simulink model "featureExtractionTest"  (R2021a)
settings: Solver=FixedStepDiscrete  StartTime=0.0  StopTime=stopTime  RelTol=1e-3
PostLoadFcn:
  | addpath([fileparts(which(bdroot)) filesep '..' filesep])
InitFcn:
  | simulinkInitFeatureExtraction
StopFcn:
  | simulinkVerifyFeatureExtraction
undefined symbols (not defined in the file or in its folder): params
libraries: hdlsllib x10, dspsrcs4 x1
settings Model: DataTypeOverride=Off  SimulationMode=accelerator  PauseTimes=1  Creator=trevor  LastModifiedBy=trevvvy
settings SolverCC: AlgebraicLoopSolver=TrustRegion
settings DataIOCC: SaveFormat=Array  SaveOutput=off  DSMLogging=off  SaveTime=off  ReturnWorkspaceOutputs=off
settings OptimizationCC: BlockReduction=off  ConditionallyExecuteInputs=off  DefaultParameterBehavior=Inlined
settings DebuggingCC: AlgebraicLoopMsg=error  SingleTaskRateTransMsg=error
settings HardwareCC: ProdBitPerPointer=32  ProdBitPerSizeT=32  ProdBitPerPtrDiffT=32  ProdLargestAtomicFloat=None  ProdIntDivRoundTo=Undefined  ProdEndianess=Unspecified  ProdWordSize=32  ProdHWDeviceType=ASIC/FPGA->ASIC/FPGA  TargetBitPerLong=64  TargetBitPerPointer=64  TargetBitPerSizeT=64  TargetBitPerPtrDiffT=64  TargetLongLongMode=on  TargetIntDivRoundTo=Zero  TargetEndianess=LittleEndian  TargetWordSize=64  TargetHWDeviceType=Custom Processor->MATLAB Host Computer  ProdEqTarget=off

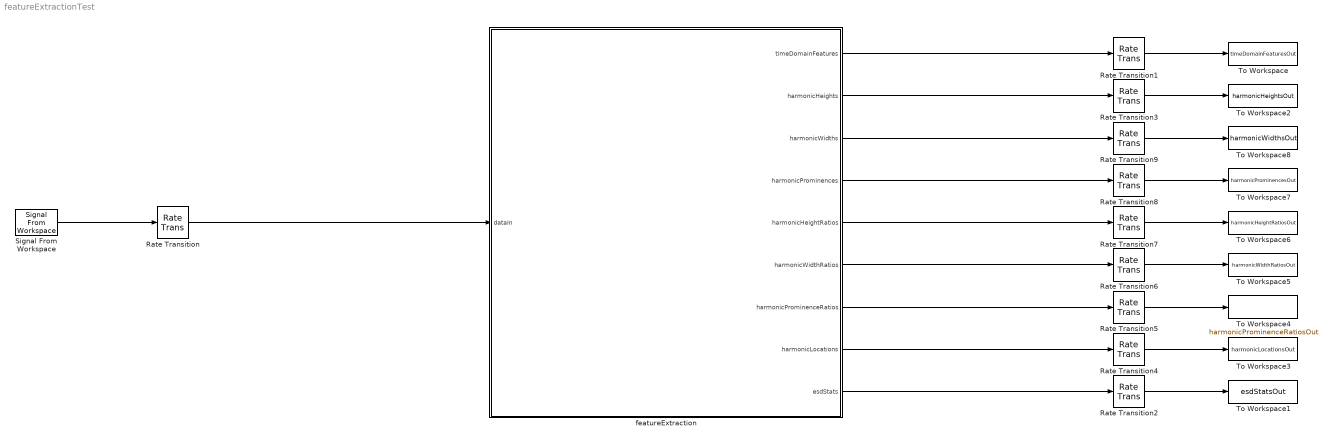
== system featureExtractionTest ==
  Rate Transition : RateTransition  Deterministic=off  OutPortSampleTime=params.systemClockPeriod
  Rate Transition{1..9} (9 alike) : RateTransition  OutPortSampleTime=params.samplingPeriod
  Signal From Workspace : dspsrcs4/Signal From Workspace  X=testData  Ts=params.samplingPeriod  nsamps=1  OutputAfterFinalValue=Setting to zero  ignoreOrWarnInputAndFrameLengths=off  OutputFrames=off
  To Workspace : ToWorkspace  VariableName=timeDomainFeaturesOut  SampleTime=-1
      settings: Save2DSignal=2-D array (concatenate along first dimension)
  To Workspace1 : ToWorkspace  VariableName=esdStatsOut  SampleTime=-1
      settings: Save2DSignal=2-D array (concatenate along first dimension)
  To Workspace2 : ToWorkspace  VariableName=harmonicHeightsOut  SampleTime=-1
      settings: Save2DSignal=2-D array (concatenate along first dimension)
  To Workspace3 : ToWorkspace  VariableName=harmonicLocationsOut  SampleTime=-1
      settings: Save2DSignal=2-D array (concatenate along first dimension)
  To Workspace4 : ToWorkspace  VariableName=harmonicProminenceRatiosOut  SampleTime=-1
      settings: Save2DSignal=2-D array (concatenate along first dimension)
  To Workspace5 : ToWorkspace  VariableName=harmonicWidthRatiosOut  SampleTime=-1
      settings: Save2DSignal=2-D array (concatenate along first dimension)
  To Workspace6 : ToWorkspace  VariableName=harmonicHeightRatiosOut  SampleTime=-1
      settings: Save2DSignal=2-D array (concatenate along first dimension)
  To Workspace7 : ToWorkspace  VariableName=harmonicProminencesOut  SampleTime=-1
      settings: Save2DSignal=2-D array (concatenate along first dimension)
  To Workspace8 : ToWorkspace  VariableName=harmonicWidthsOut  SampleTime=-1
      settings: Save2DSignal=2-D array (concatenate along first dimension)
  featureExtraction : Subsystem
  wires:
  Signal From Workspace/1 -> Rate Transition/1
  Rate Transition1/1 -> To Workspace/1
  Rate Transition2/1 -> To Workspace1/1
  Rate Transition3/1 -> To Workspace2/1
  Rate Transition4/1 -> To Workspace3/1
  Rate Transition5/1 -> To Workspace4/1
  Rate Transition6/1 -> To Workspace5/1
  Rate Transition7/1 -> To Workspace6/1
  Rate Transition9/1 -> To Workspace8/1
  Rate Transition8/1 -> To Workspace7/1
  Rate Transition/1 -> featureExtraction/1(dataIn)
  featureExtraction/1(timeDomainFeatures) -> Rate Transition1/1
  featureExtraction/2(harmonicHeights) -> Rate Transition3/1
  featureExtraction/3(harmonicWidths) -> Rate Transition9/1
  featureExtraction/4(harmonicProminences) -> Rate Transition8/1
  featureExtraction/5(harmonicHeightRatios) -> Rate Transition7/1
  featureExtraction/6(harmonicWidthRatios) -> Rate Transition6/1
  featureExtraction/7(harmonicProminenceRatios) -> Rate Transition5/1
  featureExtraction/8(harmonicLocations) -> Rate Transition4/1
  featureExtraction/9(esdStats) -> Rate Transition2/1

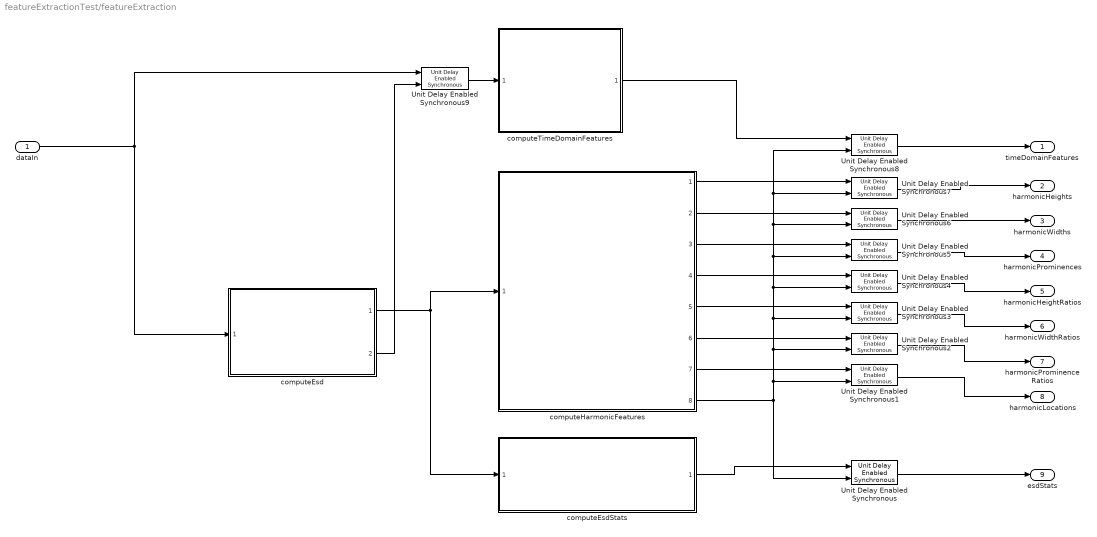
== system featureExtractionTest/featureExtraction ==
  dataIn : Inport
  Unit Delay Enabled Synchronous{,1..9} (10 alike) : hdlsllib/Discrete/Unit Delay Enabled Synchronous  InitialCondition=0.0  SampleTime=-1
      settings: SourceProductBaseCode=SL
  computeEsd : Subsystem  ReferencedSubsystem=ESD
  computeEsdStats : Subsystem  ReferencedSubsystem=extractEsdStats
  computeHarmonicFeatures : Subsystem  ReferencedSubsystem=harmonicFeatures
  computeTimeDomainFeatures : Subsystem  ReferencedSubsystem=timeDomainFeatures
  timeDomainFeatures : Outport
  harmonicHeights : Outport  Port=2
  harmonicWidths : Outport  Port=3
  harmonicProminences : Outport  Port=4
  harmonicHeightRatios : Outport  Port=5
  harmonicWidthRatios : Outport  Port=6
  harmonicProminenceRatios : Outport  Port=7
  harmonicLocations : Outport  Port=8
  esdStats : Outport  Port=9
  wires:
  computeHarmonicFeatures/6 -> Unit Delay Enabled Synchronous2/1
  Unit Delay Enabled Synchronous3/1 -> harmonicWidthRatios/1
  Unit Delay Enabled Synchronous8/1 -> timeDomainFeatures/1
  computeEsd/1 -> computeEsdStats/1, computeHarmonicFeatures/1
  computeTimeDomainFeatures/1 -> Unit Delay Enabled Synchronous8/1
  computeHarmonicFeatures/7 -> Unit Delay Enabled Synchronous1/1
  computeHarmonicFeatures/5 -> Unit Delay Enabled Synchronous3/1
  dataIn/1 -> computeEsd/1, Unit Delay Enabled Synchronous9/1
  Unit Delay Enabled Synchronous7/1 -> harmonicHeights/1
  computeEsdStats/1 -> Unit Delay Enabled Synchronous/1
  Unit Delay Enabled Synchronous/1 -> esdStats/1
  Unit Delay Enabled Synchronous5/1 -> harmonicProminences/1
  Unit Delay Enabled Synchronous6/1 -> harmonicWidths/1
  Unit Delay Enabled Synchronous4/1 -> harmonicHeightRatios/1
  Unit Delay Enabled Synchronous2/1 -> harmonicProminenceRatios/1
  computeHarmonicFeatures/3 -> Unit Delay Enabled Synchronous5/1
  computeHarmonicFeatures/2 -> Unit Delay Enabled Synchronous6/1
  computeHarmonicFeatures/8 -> Unit Delay Enabled Synchronous/2, Unit Delay Enabled Synchronous8/2, Unit Delay Enabled Synchronous7/2, Unit Delay Enabled Synchronous6/2, Unit Delay Enabled Synchronous5/2, Unit Delay Enabled Synchronous4/2, Unit Delay Enabled Synchronous3/2, Unit Delay Enabled Synchronous2/2, Unit Delay Enabled Synchronous1/2
  computeHarmonicFeatures/4 -> Unit Delay Enabled Synchronous4/1
  computeEsd/2 -> Unit Delay Enabled Synchronous9/2
  Unit Delay Enabled Synchronous1/1 -> harmonicLocations/1
  Unit Delay Enabled Synchronous9/1 -> computeTimeDomainFeatures/1
  computeHarmonicFeatures/1 -> Unit Delay Enabled Synchronous7/1
